simulink model "New_Boom_Controller"  (R2020a)
settings: Solver=VariableStepAuto  StartTime=0.0  StopTime=30  RelTol=1e-3
values from neighbouring files (symbols this model uses):
  Bm = 4    [Boom_Control.m]
  Jm = 0.2    [Boom_Control.m]
  Kd = 0    [Boom_Control.m]
  Ke = 1.2    [Boom_Control.m]
  Kp = 10    [Boom_Control.m]
  Kt = 1.5    [Boom_Control.m]
  La = 0.001    [Boom_Control.m]
  Ra = 0.3    [Boom_Control.m]
  TL = 0.8    [Boom_Control.m]
libraries: simulink_extras x2
settings Model: Creator=alan  LastModifiedBy=alan

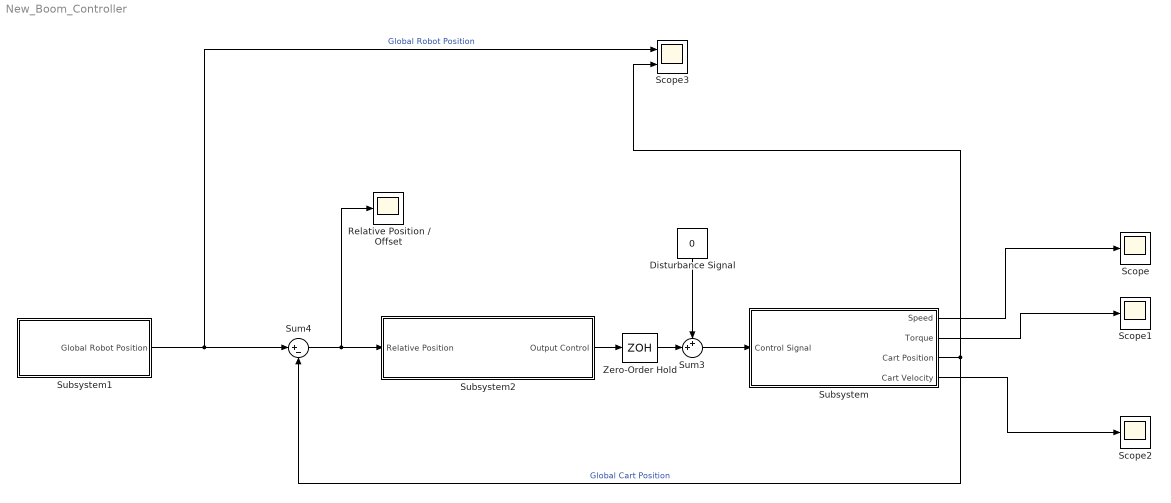
== system New_Boom_Controller ==
  Disturbance Signal : Constant  Value=0
  Relative Position / Offset : Scope
  Scope : Scope
  Scope1 : Scope
  Scope2 : Scope
  Scope3 : Scope  NumInputPorts=2
  Subsystem : Subsystem
  Subsystem1 : Subsystem
  Subsystem2 : Subsystem
  Sum3 : Sum  Inputs=++|
  Sum4 : Sum  Inputs=|+-
  Zero-Order Hold : ZeroOrderHold  SampleTime=0.01
  wires:
  Disturbance Signal/1 -> Sum3/1
  Subsystem/3(Cart Position) -> Scope3/2, Sum4/2  "Global Cart Position"
  Subsystem/1(Speed) -> Scope/1
  Sum3/1 -> Subsystem/1(Control Signal)
  Subsystem/2(Torque) -> Scope1/1
  Subsystem/4(Cart Velocity) -> Scope2/1
  Subsystem1/1(Global Robot Position) -> Scope3/1, Sum4/1  "Global Robot Position"
  Sum4/1 -> Relative Position / Offset/1, Subsystem2/1(Relative Position)
  Subsystem2/1(Output Control) -> Zero-Order Hold/1
  Zero-Order Hold/1 -> Sum3/2

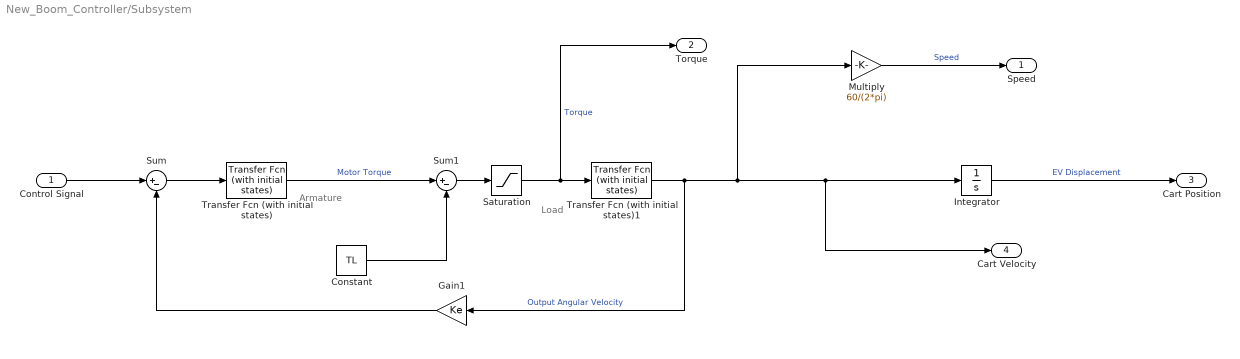
== system New_Boom_Controller/Subsystem ==
  note: Load
  note: Armature
  Control Signal : Inport
  Constant : Constant  Value=TL
  Gain1 : Gain  Gain=Ke
  Integrator : Integrator
  Multiply : Gain  Gain=60/(2*pi)
  Saturation : Saturate  UpperLimit=2  LowerLimit=-2
  Sum : Sum  Inputs=|+-
  Sum1 : Sum  Inputs=|+-
  Transfer Fcn (with initial states) : simulink_extras/Additional Linear/Transfer Fcn (with initial states)  N=Kt  D="[La  Ra]"  X0=0
  Transfer Fcn (with initial states)1 : simulink_extras/Additional Linear/Transfer Fcn (with initial states)  N=1  D="[Jm  Bm]"  X0=0
  Speed : Outport
  Torque : Outport  Port=2
  Cart Position : Outport  Port=3
  Cart Velocity : Outport  Port=4
  wires:
  Transfer Fcn (with initial states)/1 -> Sum1/1  "Motor Torque"
  Sum1/1 -> Saturation/1
  Transfer Fcn (with initial states)1/1 -> Integrator/1, Cart Velocity/1, Multiply/1, Gain1/1  "Output Angular Velocity"
  Saturation/1 -> Torque/1, Transfer Fcn (with initial states)1/1  "Torque"
  Multiply/1 -> Speed/1  "Speed"
  Gain1/1 -> Sum/2
  Sum/1 -> Transfer Fcn (with initial states)/1
  Constant/1 -> Sum1/2
  Integrator/1 -> Cart Position/1  "EV Displacement"
  Control Signal/1 -> Sum/1

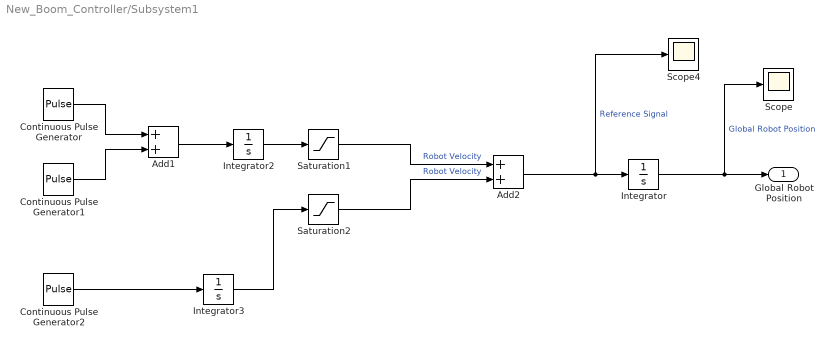
== system New_Boom_Controller/Subsystem1 ==
  Add1 : Sum
  Add2 : Sum
  Continuous Pulse Generator : DiscretePulseGenerator  PulseType=Time based  Amplitude=0.2  Period=5  PulseWidth=50
  Continuous Pulse Generator1 : DiscretePulseGenerator  PulseType=Time based  Amplitude=-0.4  Period=5  PulseWidth=50  PhaseDelay=5
  Continuous Pulse Generator2 : DiscretePulseGenerator  PulseType=Time based  Amplitude=0.2  Period=5  PulseWidth=50  PhaseDelay=15
  Integrator : Integrator
  Integrator2 : Integrator
  Integrator3 : Integrator
  Saturation1 : Saturate  UpperLimit=2
  Saturation2 : Saturate  UpperLimit=.5
  Scope : Scope
  Scope4 : Scope
  Global Robot Position : Outport
  wires:
  Integrator3/1 -> Saturation2/1
  Integrator2/1 -> Saturation1/1
  Continuous Pulse Generator/1 -> Add1/1
  Saturation2/1 -> Add2/2  "Robot Velocity"
  Continuous Pulse Generator2/1 -> Integrator3/1
  Add2/1 -> Integrator/1, Scope4/1  "Reference Signal"
  Saturation1/1 -> Add2/1  "Robot Velocity"
  Continuous Pulse Generator1/1 -> Add1/2
  Add1/1 -> Integrator2/1
  Integrator/1 -> Scope/1, Global Robot Position/1  "Global Robot Position"

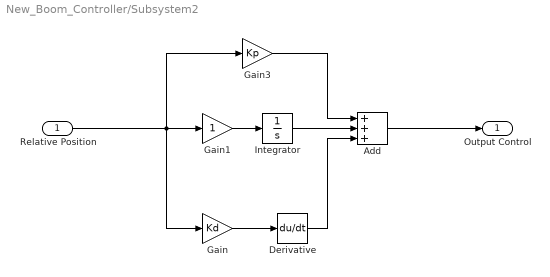
== system New_Boom_Controller/Subsystem2 ==
  Relative Position : Inport
  Add : Sum  Inputs=+++
  Derivative : Derivative
  Gain : Gain  Gain=Kd
  Gain1 : Gain
  Gain3 : Gain  Gain=Kp
  Integrator : Integrator
  Output Control : Outport
  wires:
  Gain/1 -> Derivative/1
  Gain3/1 -> Add/1
  Derivative/1 -> Add/3
  Add/1 -> Output Control/1
  Relative Position/1 -> Gain1/1, Gain/1, Gain3/1
  Gain1/1 -> Integrator/1
  Integrator/1 -> Add/2
